simulink model "ZadacaII48"  (R2021a)
settings: Solver=VariableStepAuto  StartTime=0.0  StopTime=3  RelTol=1e-3
settings Model: Creator=stojo  LastModifiedBy=stojo

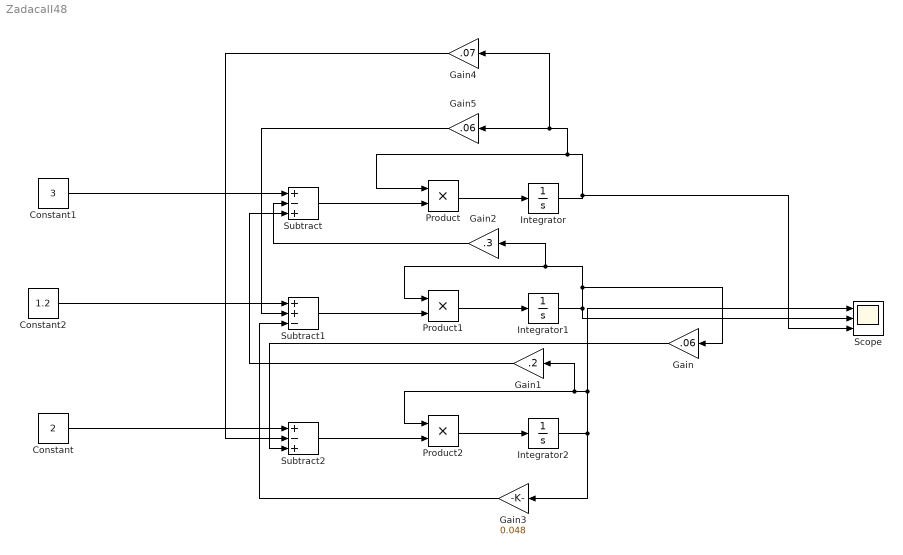
== system ZadacaII48 ==
  Constant : Constant  Value=2
  Constant1 : Constant  Value=3
  Constant2 : Constant  Value=1.2
  Gain : Gain  Gain=.06
  Gain1 : Gain  Gain=.2
  Gain2 : Gain  Gain=.3
  Gain3 : Gain  Gain=0.048
  Gain4 : Gain  Gain=.07
  Gain5 : Gain  Gain=.06
  Integrator : Integrator  InitialCondition=8
  Integrator1 : Integrator  InitialCondition=6
  Integrator2 : Integrator  InitialCondition=5
  Product : Product
  Product1 : Product
  Product2 : Product
  Scope : Scope  NumInputPorts=3
  Subtract : Sum  Inputs=+-+
  Subtract1 : Sum  Inputs=++-
  Subtract2 : Sum  Inputs=+-+
  wires:
  Subtract1/1 -> Product1/2
  Subtract2/1 -> Product2/2
  Product2/1 -> Integrator2/1
  Integrator2/1 -> Scope/1, Gain1/1, Product2/1, Gain3/1
  Product1/1 -> Integrator1/1
  Integrator1/1 -> Scope/2, Gain/1, Gain2/1, Product1/1
  Product/1 -> Integrator/1
  Subtract/1 -> Product/2
  Integrator/1 -> Scope/3, Gain4/1, Gain5/1, Product/1
  Constant/1 -> Subtract2/1
  Constant2/1 -> Subtract1/1
  Constant1/1 -> Subtract/1
  Gain2/1 -> Subtract/2
  Gain1/1 -> Subtract/3
  Gain/1 -> Subtract2/3
  Gain3/1 -> Subtract1/3
  Gain5/1 -> Subtract1/2
  Gain4/1 -> Subtract2/2
